simulink model "stf_pro_1"  (R2024b)
settings: Solver=VariableStepAuto  StartTime=0.0  StopTime=inf  RelTol=1e-3
settings Model: Creator=hp  LastModifiedBy=hp

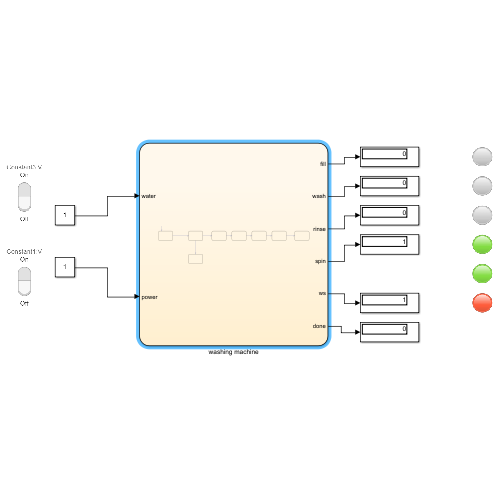
[thumbnail: Simulink's stored preview of the top-level diagram]
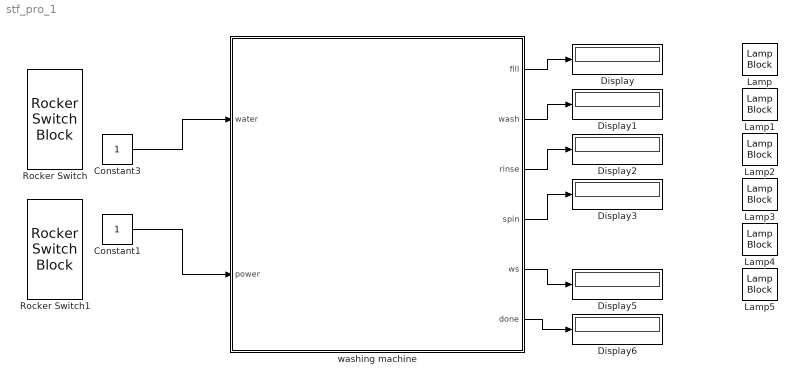
== system stf_pro_1 ==
  Constant1 : Constant
  Constant3 : Constant
  Display{,1..3,5..6} (6 alike) : Display
  Lamp{,1..5} (6 alike) : LampBlock  LabelPosition=Hide
  Rocker Switch : RockerSwitchBlock
      settings: Values={{'Off', 'On'}, [0 1]}
  Rocker Switch1 : RockerSwitchBlock
      settings: Values={{'Off', 'On'}, [0 1]}
  washing machine : Stateflow chart  TreatAsAtomicUnit=on
  wires:
  Constant3/1 -> washing machine/1(water)
  Constant1/1 -> washing machine/2(power)
  washing machine/1(fill) -> Display/1
  washing machine/2(wash) -> Display1/1
  washing machine/3(rinse) -> Display2/1
  washing machine/4(spin) -> Display3/1
  washing machine/5(ws) -> Display5/1
  washing machine/6(done) -> Display6/1

== stateflow chart stf_pro_1/washing machine ==
  state power_supply
  state water_supply
  state fill
    entry:
    fill=1;
  state wash
    entry:
    fill=0,wash=1;
  state rinse
    entry:
    wash=0,rinse=1;
  state spin
    entry:
    rinse=0,spin=1;
  state done
    entry:
    spin=0,done=1;
  state water_indicator
    entry:
    ws=1;
  (default) -> power_supply
  power_supply -> water_supply : [power==1]
  water_supply -> fill [order 1] : [water==1]
  fill -> wash : after(10,sec)
  wash -> rinse : after(10,sec)
  rinse -> spin : after(10,sec)
  spin -> done : after(10,sec)
  water_supply -> water_indicator [order 2] : [water==1]
  data: water input; fill output; wash output; rinse output; spin output; ws output; done output; power input
